simulink model "capitol4pb1"  (R2013a)
settings: Solver=ode45  StartTime=0.0  StopTime=500  RelTol=1e-3
undefined symbols (not defined in the file): des, gcbh
settings Model: Creator=user  LastModifiedBy=user

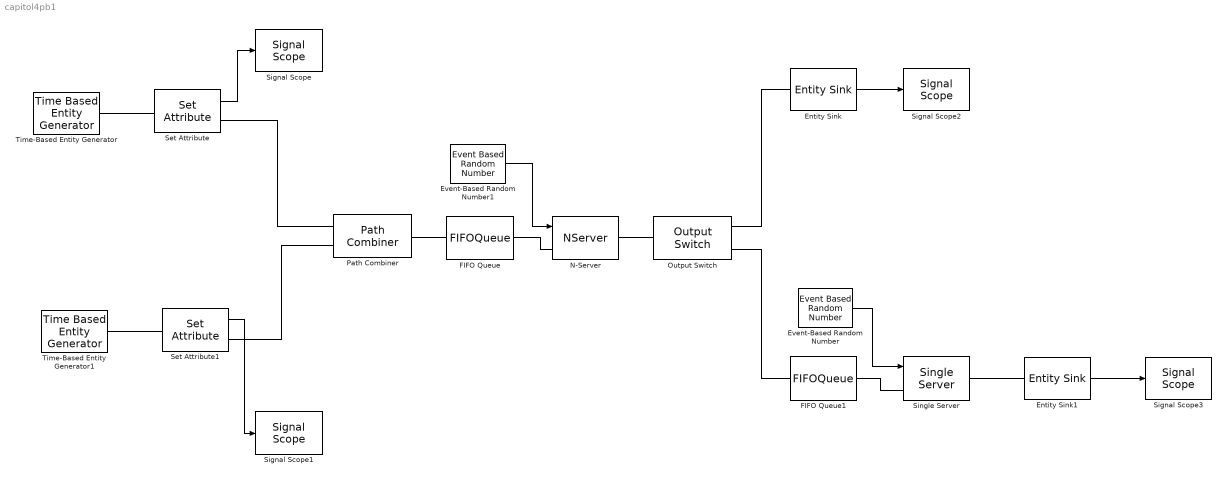
== system capitol4pb1 ==
  Entity Sink : EntitySink  StatNumberArrived=on
  Entity Sink1 : EntitySink  StatNumberArrived=on
  Event-Based Random Number : EventBasedRandomNumber  Distribution=Uniform  minUnif=8  maxUnif=12
  Event-Based Random Number1 : EventBasedRandomNumber  Distribution=Uniform  minUnif=14  maxUnif=22
  FIFO Queue : FIFOQueue
  FIFO Queue1 : FIFOQueue
  N-Server : NServer  NumberOfServers=2  ServiceTimeFrom=Signal port t
  Output Switch : OutputSwitch  NumberOutputPorts=2  SwitchingCriterion=From attribute
  Path Combiner : PathCombiner  NumberInputPorts=2
  Set Attribute : SetAttribute  StatNumberDeparted=on  EvaluatedAttributeValue={ 1}
  Set Attribute1 : SetAttribute  AttributeValue=2  StatNumberDeparted=on  EvaluatedAttributeValue={ 2}
  Signal Scope : SignalScope  LoadFcn=des.scope.CallbackSupport('seLoadFcn',gcbh)  StartFcn=des.scope.CallbackSupport('seStartFcn',gcbh)  StopFcn=des.scope.CallbackSupport('seStopFcn',gcbh)
      settings: CopyFcn=des.scope.CallbackSupport('seCopyFcn',gcbh)  DeleteFcn=des.scope.CallbackSupport('seDeleteFcn',gcbh)  PreSaveFcn=des.scope.CallbackSupport('sePreSaveFcn',gcbh)  NameChangeFcn=des.scope.CallbackSupport('seNameChangeFcn',gcbh)  OpenFcn=des.scope.CallbackSupport('seOpenFcn',gcbh)
  Signal Scope1 : SignalScope  LoadFcn=des.scope.CallbackSupport('seLoadFcn',gcbh)  StartFcn=des.scope.CallbackSupport('seStartFcn',gcbh)  StopFcn=des.scope.CallbackSupport('seStopFcn',gcbh)
      settings: CopyFcn=des.scope.CallbackSupport('seCopyFcn',gcbh)  DeleteFcn=des.scope.CallbackSupport('seDeleteFcn',gcbh)  PreSaveFcn=des.scope.CallbackSupport('sePreSaveFcn',gcbh)  NameChangeFcn=des.scope.CallbackSupport('seNameChangeFcn',gcbh)  OpenFcn=des.scope.CallbackSupport('seOpenFcn',gcbh)
  Signal Scope2 : SignalScope  LoadFcn=des.scope.CallbackSupport('seLoadFcn',gcbh)  StartFcn=des.scope.CallbackSupport('seStartFcn',gcbh)  StopFcn=des.scope.CallbackSupport('seStopFcn',gcbh)  XMax=640
      settings: CopyFcn=des.scope.CallbackSupport('seCopyFcn',gcbh)  DeleteFcn=des.scope.CallbackSupport('seDeleteFcn',gcbh)  PreSaveFcn=des.scope.CallbackSupport('sePreSaveFcn',gcbh)  NameChangeFcn=des.scope.CallbackSupport('seNameChangeFcn',gcbh)  OpenFcn=des.scope.CallbackSupport('seOpenFcn',gcbh)  YMax=20
  Signal Scope3 : SignalScope  LoadFcn=des.scope.CallbackSupport('seLoadFcn',gcbh)  StartFcn=des.scope.CallbackSupport('seStartFcn',gcbh)  StopFcn=des.scope.CallbackSupport('seStopFcn',gcbh)
      settings: CopyFcn=des.scope.CallbackSupport('seCopyFcn',gcbh)  DeleteFcn=des.scope.CallbackSupport('seDeleteFcn',gcbh)  PreSaveFcn=des.scope.CallbackSupport('sePreSaveFcn',gcbh)  NameChangeFcn=des.scope.CallbackSupport('seNameChangeFcn',gcbh)  OpenFcn=des.scope.CallbackSupport('seOpenFcn',gcbh)
  Single Server : SingleServer  ServiceTimeFrom=Signal port t
  Time-Based Entity Generator : TimeBasedEntityGenerator  Distribution=Uniform  Minimum=25  Maximum=45
  Time-Based Entity Generator1 : TimeBasedEntityGenerator  Distribution=Uniform  Minimum=38  Maximum=52
  wires:
  Entity Sink/1 -> Signal Scope2/1
  Entity Sink1/1 -> Signal Scope3/1
  Event-Based Random Number/1 -> Single Server/1
  Set Attribute1/1 -> Signal Scope1/1
  Set Attribute/1 -> Signal Scope/1
  Event-Based Random Number1/1 -> N-Server/1
  connections:
  Single Server/RConn1 -- Entity Sink1/LConn1
  FIFO Queue1/RConn1 -- Single Server/LConn1
  Output Switch/RConn1 -- Entity Sink/LConn1
  Output Switch/RConn2 -- FIFO Queue1/LConn1
  N-Server/RConn1 -- Output Switch/LConn1
  FIFO Queue/RConn1 -- N-Server/LConn1
  Path Combiner/RConn1 -- FIFO Queue/LConn1
  Set Attribute1/RConn1 -- Path Combiner/LConn2
  Set Attribute/RConn1 -- Path Combiner/LConn1
  Time-Based Entity Generator/RConn1 -- Set Attribute/LConn1
  Time-Based Entity Generator1/RConn1 -- Set Attribute1/LConn1
